simulink model "case6"  (R2024b)
settings: Solver=FixedStepAuto  StartTime=0  StopTime=1  FixedStep=1e-7  RelTol=1e-3
values from neighbouring files (symbols this model uses):
  SG_D_1_D = 0.01056    [IEEE9_case_parameters.m]    (also in case1_parameters.m; case2_parameters.m; case3_parameters.m; case4_parameters.m)
  SG_D_1_EnableSaturation = 0    [IEEE9_case_parameters.m]    (also in case1_parameters.m; case2_parameters.m; case3_parameters.m; case4_parameters.m)
  SG_D_1_f0 = 60    [IEEE9_case_parameters.m]    (also in case1_parameters.m; case2_parameters.m; case3_parameters.m; case4_parameters.m)
  SG_D_1_H = 7.5    [IEEE9_case_parameters.m]    (also in case1_parameters.m; case2_parameters.m; case3_parameters.m; case4_parameters.m)
  SG_D_1_K_A = 20    [IEEE9_case_parameters.m]    (also in case1_parameters.m; case2_parameters.m; case3_parameters.m; case4_parameters.m)
  SG_D_1_K_E = 1.000000e+1    (= 10)    [IEEE9_case_parameters.m]    (also in case1_parameters.m; case2_parameters.m; case3_parameters.m; case4_parameters.m)
  SG_D_1_K_F = 2.363    [IEEE9_case_parameters.m]    (also in case1_parameters.m; case2_parameters.m; case3_parameters.m; case4_parameters.m)
  SG_D_1_K_s = 0.5    [IEEE9_case_parameters.m]    (also in case1_parameters.m = 5; case2_parameters.m = 5; case3_parameters.m = 5; case4_parameters.m = 5)
  SG_D_1_R_a = 0.001088    [IEEE9_case_parameters.m]    (also in case1_parameters.m; case2_parameters.m; case3_parameters.m; case4_parameters.m)
  SG_D_1_S_A = 1    [IEEE9_case_parameters.m]    (also in case1_parameters.m; case2_parameters.m; case3_parameters.m; case4_parameters.m)
  SG_D_1_S_B = 0.103    [IEEE9_case_parameters.m]    (also in case1_parameters.m; case2_parameters.m; case3_parameters.m; case4_parameters.m)
  SG_D_1_S_N = 10.659857    [IEEE9_case_parameters.m]    (also in case1_parameters.m; case2_parameters.m; case3_parameters.m; case4_parameters.m)
  SG_D_1_SpeedPara = 200    [IEEE9_case_parameters.m]    (also in case1_parameters.m; case2_parameters.m; case3_parameters.m; case4_parameters.m)
  SG_D_1_T_0 = 0.720173    [IEEE9_case_parameters.m]    (also in case1_parameters.m = 0.755522; case2_parameters.m = 0.808931; case3_parameters.m = 0.869402; case4_parameters.m = 0.729316)
  SG_D_1_T_1 = 0.3    [IEEE9_case_parameters.m]    (also in case1_parameters.m; case2_parameters.m; case3_parameters.m; case4_parameters.m)
  SG_D_1_T_2 = 0.05    [IEEE9_case_parameters.m]    (also in case1_parameters.m; case2_parameters.m; case3_parameters.m; case4_parameters.m)
  SG_D_1_T_3 = 0.02    [IEEE9_case_parameters.m]    (also in case1_parameters.m; case2_parameters.m; case3_parameters.m; case4_parameters.m)
  SG_D_1_T_4 = 0.005    [IEEE9_case_parameters.m]    (also in case1_parameters.m; case2_parameters.m; case3_parameters.m; case4_parameters.m)
  SG_D_1_T_A = 0.02    [IEEE9_case_parameters.m]    (also in case1_parameters.m; case2_parameters.m; case3_parameters.m; case4_parameters.m)
  SG_D_1_T_dd = 8.000000e+0    (= 8)    [IEEE9_case_parameters.m]    (also in case1_parameters.m; case2_parameters.m; case3_parameters.m; case4_parameters.m)
  SG_D_1_T_ddd = 0.04    [IEEE9_case_parameters.m]    (also in case1_parameters.m; case2_parameters.m; case3_parameters.m; case4_parameters.m)
  SG_D_1_T_E = 0.314    [IEEE9_case_parameters.m]    (also in case1_parameters.m; case2_parameters.m; case3_parameters.m; case4_parameters.m)
  SG_D_1_T_F = 0.35    [IEEE9_case_parameters.m]    (also in case1_parameters.m; case2_parameters.m; case3_parameters.m; case4_parameters.m)
  SG_D_1_T_qd = 0.8    [IEEE9_case_parameters.m]    (also in case1_parameters.m; case2_parameters.m; case3_parameters.m; case4_parameters.m)
  SG_D_1_T_qdd = 0.02    [IEEE9_case_parameters.m]    (also in case1_parameters.m; case2_parameters.m; case3_parameters.m; case4_parameters.m)
  SG_D_1_T_speed = 0.1    [IEEE9_case_parameters.m]    (also in case1_parameters.m = 200; case2_parameters.m = 200; case3_parameters.m = 200; case4_parameters.m = 200)
  SG_D_1_T_w = 0.5    [IEEE9_case_parameters.m]    (also in case1_parameters.m; case2_parameters.m; case3_parameters.m; case4_parameters.m)
  SG_D_1_V_ref = 1.990276    [IEEE9_case_parameters.m]    (also in case1_parameters.m = 2.042296; case2_parameters.m = 2.051388; case3_parameters.m = 2.089584; case4_parameters.m = 2.01845)
  SG_D_1_w_ref = 376.991118    [IEEE9_case_parameters.m]    (also in case1_parameters.m; case2_parameters.m; case3_parameters.m; case4_parameters.m)
  SG_D_1_wb = 6.000000e+1    (= 60)    [IEEE9_case_parameters.m]    (also in case1_parameters.m; case2_parameters.m; case3_parameters.m; case4_parameters.m)
  SG_D_1_x_d = 1.9    [IEEE9_case_parameters.m]    (also in case1_parameters.m; case2_parameters.m; case3_parameters.m; case4_parameters.m)
  SG_D_1_x_dd = 0.302    [IEEE9_case_parameters.m]    (also in case1_parameters.m; case2_parameters.m; case3_parameters.m; case4_parameters.m)
  SG_D_1_x_ddd = 0.204    [IEEE9_case_parameters.m]    (also in case1_parameters.m; case2_parameters.m; case3_parameters.m; case4_parameters.m)
  SG_D_1_x_l = 0.05    [IEEE9_case_parameters.m]    (also in case1_parameters.m; case2_parameters.m; case3_parameters.m; case4_parameters.m)
  SG_D_1_x_q = 1.3    [IEEE9_case_parameters.m]    (also in case1_parameters.m; case2_parameters.m; case3_parameters.m; case4_parameters.m)
  SG_D_1_x_qd = 0.5    [IEEE9_case_parameters.m]    (also in case1_parameters.m; case2_parameters.m; case3_parameters.m; case4_parameters.m)
  SG_D_1_x_qdd = 0.3    [IEEE9_case_parameters.m]    (also in case1_parameters.m; case2_parameters.m; case3_parameters.m; case4_parameters.m)
  SG_D_2_D = 0.02    [IEEE9_case_parameters.m]    (also in case1_parameters.m; case2_parameters.m; case3_parameters.m; case4_parameters.m)
  SG_D_2_EnableSaturation = 0    [IEEE9_case_parameters.m]    (also in case1_parameters.m; case2_parameters.m; case3_parameters.m; case4_parameters.m)
  SG_D_2_f0 = 60    [IEEE9_case_parameters.m]    (also in case1_parameters.m; case2_parameters.m; case3_parameters.m; case4_parameters.m)
  SG_D_2_H = 8.000000e+0    (= 8)    [IEEE9_case_parameters.m]    (also in case1_parameters.m; case2_parameters.m; case3_parameters.m; case4_parameters.m)
  SG_D_2_K_A = 20    [IEEE9_case_parameters.m]    (also in case1_parameters.m; case2_parameters.m; case3_parameters.m; case4_parameters.m)
  SG_D_2_K_E = 1.000000e+1    (= 10)    [IEEE9_case_parameters.m]    (also in case1_parameters.m; case2_parameters.m; case3_parameters.m; case4_parameters.m)
  SG_D_2_K_F = 2.363    [IEEE9_case_parameters.m]    (also in case1_parameters.m; case2_parameters.m; case3_parameters.m; case4_parameters.m)
  SG_D_2_K_s = 0.5    [IEEE9_case_parameters.m]    (also in case1_parameters.m = 4; case2_parameters.m = 4; case3_parameters.m = 4; case4_parameters.m = 4)
  SG_D_2_R_a = 0.001088    [IEEE9_case_parameters.m]    (also in case1_parameters.m; case2_parameters.m; case3_parameters.m; case4_parameters.m)
  SG_D_2_S_A = 1    [IEEE9_case_parameters.m]    (also in case1_parameters.m; case2_parameters.m; case3_parameters.m; case4_parameters.m)
  SG_D_2_S_B = 0.103    [IEEE9_case_parameters.m]    (also in case1_parameters.m; case2_parameters.m; case3_parameters.m; case4_parameters.m)
  SG_D_2_S_N = 10.659857    [IEEE9_case_parameters.m]    (also in case1_parameters.m; case2_parameters.m; case3_parameters.m; case4_parameters.m)
  SG_D_2_SpeedPara = 200    [IEEE9_case_parameters.m]    (also in case1_parameters.m; case2_parameters.m; case3_parameters.m; case4_parameters.m)
  SG_D_2_T_0 = 1.632913    [IEEE9_case_parameters.m]    (also in case1_parameters.m = 1.632925; case2_parameters.m = 1.632915; case3_parameters.m = 1.632914; case4_parameters.m = 1.632927)
  SG_D_2_T_1 = 0.2    [IEEE9_case_parameters.m]    (also in case1_parameters.m; case2_parameters.m; case3_parameters.m; case4_parameters.m)
  SG_D_2_T_2 = 0.05    [IEEE9_case_parameters.m]    (also in case1_parameters.m; case2_parameters.m; case3_parameters.m; case4_parameters.m)
  SG_D_2_T_3 = 0.02    [IEEE9_case_parameters.m]    (also in case1_parameters.m; case2_parameters.m; case3_parameters.m; case4_parameters.m)
  SG_D_2_T_4 = 0.005    [IEEE9_case_parameters.m]    (also in case1_parameters.m; case2_parameters.m; case3_parameters.m; case4_parameters.m)
  SG_D_2_T_A = 0.02    [IEEE9_case_parameters.m]    (also in case1_parameters.m; case2_parameters.m; case3_parameters.m; case4_parameters.m)
  SG_D_2_T_dd = 7.9    [IEEE9_case_parameters.m]    (also in case1_parameters.m; case2_parameters.m; case3_parameters.m; case4_parameters.m)
  SG_D_2_T_ddd = 0.04    [IEEE9_case_parameters.m]    (also in case1_parameters.m; case2_parameters.m; case3_parameters.m; case4_parameters.m)
  SG_D_2_T_E = 0.314    [IEEE9_case_parameters.m]    (also in case1_parameters.m; case2_parameters.m; case3_parameters.m; case4_parameters.m)
  SG_D_2_T_F = 0.35    [IEEE9_case_parameters.m]    (also in case1_parameters.m; case2_parameters.m; case3_parameters.m; case4_parameters.m)
  SG_D_2_T_qd = 0.8    [IEEE9_case_parameters.m]    (also in case1_parameters.m; case2_parameters.m; case3_parameters.m; case4_parameters.m)
  SG_D_2_T_qdd = 0.015    [IEEE9_case_parameters.m]    (also in case1_parameters.m; case2_parameters.m; case3_parameters.m; case4_parameters.m)
  SG_D_2_T_speed = 0.1    [IEEE9_case_parameters.m]    (also in case1_parameters.m = 150; case2_parameters.m = 150; case3_parameters.m = 150; case4_parameters.m = 150)
  SG_D_2_T_w = 0.35    [IEEE9_case_parameters.m]    (also in case1_parameters.m; case2_parameters.m; case3_parameters.m; case4_parameters.m)
  SG_D_2_V_ref = 2.58547    [IEEE9_case_parameters.m]    (also in case1_parameters.m = 2.597896; case2_parameters.m = 2.587136; case3_parameters.m = 2.586042; case4_parameters.m = 2.599679)
  SG_D_2_w_ref = 376.991118    [IEEE9_case_parameters.m]    (also in case1_parameters.m; case2_parameters.m; case3_parameters.m; case4_parameters.m)
  SG_D_2_wb = 6.000000e+1    (= 60)    [IEEE9_case_parameters.m]    (also in case1_parameters.m; case2_parameters.m; case3_parameters.m; case4_parameters.m)
  SG_D_2_x_d = 1.8    [IEEE9_case_parameters.m]    (also in case1_parameters.m; case2_parameters.m; case3_parameters.m; case4_parameters.m)
  SG_D_2_x_dd = 0.302    [IEEE9_case_parameters.m]    (also in case1_parameters.m; case2_parameters.m; case3_parameters.m; case4_parameters.m)
  SG_D_2_x_ddd = 0.204    [IEEE9_case_parameters.m]    (also in case1_parameters.m; case2_parameters.m; case3_parameters.m; case4_parameters.m)
  SG_D_2_x_l = 0.05    [IEEE9_case_parameters.m]    (also in case1_parameters.m; case2_parameters.m; case3_parameters.m; case4_parameters.m)
  SG_D_2_x_q = 1.25    [IEEE9_case_parameters.m]    (also in case1_parameters.m; case2_parameters.m; case3_parameters.m; case4_parameters.m)
  SG_D_2_x_qd = 0.5    [IEEE9_case_parameters.m]    (also in case1_parameters.m; case2_parameters.m; case3_parameters.m; case4_parameters.m)
  SG_D_2_x_qdd = 0.3    [IEEE9_case_parameters.m]    (also in case1_parameters.m; case2_parameters.m; case3_parameters.m; case4_parameters.m)
  SG_D_3_D = 0.02    [IEEE9_case_parameters.m]    (also in case1_parameters.m; case2_parameters.m; case3_parameters.m; case4_parameters.m)
  SG_D_3_EnableSaturation = 0    [IEEE9_case_parameters.m]    (also in case1_parameters.m; case2_parameters.m; case3_parameters.m; case4_parameters.m)
  SG_D_3_f0 = 60    [IEEE9_case_parameters.m]    (also in case1_parameters.m; case2_parameters.m; case3_parameters.m; case4_parameters.m)
  SG_D_3_H = 7.7    [IEEE9_case_parameters.m]    (also in case1_parameters.m; case2_parameters.m; case3_parameters.m; case4_parameters.m)
  SG_D_3_K_A = 20    [IEEE9_case_parameters.m]    (also in case1_parameters.m; case2_parameters.m; case3_parameters.m; case4_parameters.m)
  SG_D_3_K_E = 1.000000e+1    (= 10)    [IEEE9_case_parameters.m]    (also in case1_parameters.m; case2_parameters.m; case3_parameters.m; case4_parameters.m)
  SG_D_3_K_F = 2.363    [IEEE9_case_parameters.m]    (also in case1_parameters.m; case2_parameters.m; case3_parameters.m; case4_parameters.m)
  SG_D_3_K_s = 0.2    [IEEE9_case_parameters.m]    (also in case1_parameters.m = 2; case2_parameters.m = 2; case3_parameters.m = 2; case4_parameters.m = 2)
  SG_D_3_R_a = 0.001088    [IEEE9_case_parameters.m]    (also in case1_parameters.m; case2_parameters.m; case3_parameters.m; case4_parameters.m)
  SG_D_3_S_A = 1    [IEEE9_case_parameters.m]    (also in case1_parameters.m; case2_parameters.m; case3_parameters.m; case4_parameters.m)
  SG_D_3_S_B = 0.103    [IEEE9_case_parameters.m]    (also in case1_parameters.m; case2_parameters.m; case3_parameters.m; case4_parameters.m)
  SG_D_3_S_N = 10.659857    [IEEE9_case_parameters.m]    (also in case1_parameters.m; case2_parameters.m; case3_parameters.m; case4_parameters.m)
  SG_D_3_SpeedPara = 200    [IEEE9_case_parameters.m]    (also in case1_parameters.m; case2_parameters.m; case3_parameters.m; case4_parameters.m)
  SG_D_3_T_0 = 0.850788    [IEEE9_case_parameters.m]    (also in case1_parameters.m = 0.850786; case2_parameters.m = 0.850787; case3_parameters.m; case4_parameters.m = 0.850786)
  SG_D_3_T_1 = 0.2    [IEEE9_case_parameters.m]    (also in case1_parameters.m; case2_parameters.m; case3_parameters.m; case4_parameters.m)
  SG_D_3_T_2 = 0.05    [IEEE9_case_parameters.m]    (also in case1_parameters.m; case2_parameters.m; case3_parameters.m; case4_parameters.m)
  SG_D_3_T_3 = 0.02    [IEEE9_case_parameters.m]    (also in case1_parameters.m; case2_parameters.m; case3_parameters.m; case4_parameters.m)
  SG_D_3_T_4 = 0.005    [IEEE9_case_parameters.m]    (also in case1_parameters.m; case2_parameters.m; case3_parameters.m; case4_parameters.m)
  SG_D_3_T_A = 0.02    [IEEE9_case_parameters.m]    (also in case1_parameters.m; case2_parameters.m; case3_parameters.m; case4_parameters.m)
  SG_D_3_T_dd = 8.1    [IEEE9_case_parameters.m]    (also in case1_parameters.m; case2_parameters.m; case3_parameters.m; case4_parameters.m)
  SG_D_3_T_ddd = 0.04    [IEEE9_case_parameters.m]    (also in case1_parameters.m; case2_parameters.m; case3_parameters.m; case4_parameters.m)
  SG_D_3_T_E = 0.314    [IEEE9_case_parameters.m]    (also in case1_parameters.m; case2_parameters.m; case3_parameters.m; case4_parameters.m)
  SG_D_3_T_F = 0.35    [IEEE9_case_parameters.m]    (also in case1_parameters.m; case2_parameters.m; case3_parameters.m; case4_parameters.m)
  SG_D_3_T_qd = 0.8    [IEEE9_case_parameters.m]    (also in case1_parameters.m; case2_parameters.m; case3_parameters.m; case4_parameters.m)
  SG_D_3_T_qdd = 0.015    [IEEE9_case_parameters.m]    (also in case1_parameters.m; case2_parameters.m; case3_parameters.m; case4_parameters.m)
  SG_D_3_T_speed = 0.1    [IEEE9_case_parameters.m]    (also in case1_parameters.m = 180; case2_parameters.m = 180; case3_parameters.m = 180; case4_parameters.m = 180)
  SG_D_3_T_w = 0.4    [IEEE9_case_parameters.m]    (also in case1_parameters.m; case2_parameters.m; case3_parameters.m; case4_parameters.m)
  SG_D_3_V_ref = 1.892727    [IEEE9_case_parameters.m]    (also in case1_parameters.m = 1.906439; case2_parameters.m = 1.895535; case3_parameters.m = 1.892105; case4_parameters.m = 1.906598)
  SG_D_3_w_ref = 376.991118    [IEEE9_case_parameters.m]    (also in case1_parameters.m; case2_parameters.m; case3_parameters.m; case4_parameters.m)
  SG_D_3_wb = 6.000000e+1    (= 60)    [IEEE9_case_parameters.m]    (also in case1_parameters.m; case2_parameters.m; case3_parameters.m; case4_parameters.m)
  SG_D_3_x_d = 1.85    [IEEE9_case_parameters.m]    (also in case1_parameters.m; case2_parameters.m; case3_parameters.m; case4_parameters.m)
  SG_D_3_x_dd = 0.302    [IEEE9_case_parameters.m]    (also in case1_parameters.m; case2_parameters.m; case3_parameters.m; case4_parameters.m)
  SG_D_3_x_ddd = 0.204    [IEEE9_case_parameters.m]    (also in case1_parameters.m; case2_parameters.m; case3_parameters.m; case4_parameters.m)
  SG_D_3_x_l = 0.05    [IEEE9_case_parameters.m]    (also in case1_parameters.m; case2_parameters.m; case3_parameters.m; case4_parameters.m)
  SG_D_3_x_q = 1.2    [IEEE9_case_parameters.m]    (also in case1_parameters.m; case2_parameters.m; case3_parameters.m; case4_parameters.m)
  SG_D_3_x_qd = 0.5    [IEEE9_case_parameters.m]    (also in case1_parameters.m; case2_parameters.m; case3_parameters.m; case4_parameters.m)
  SG_D_3_x_qdd = 0.3    [IEEE9_case_parameters.m]    (also in case1_parameters.m; case2_parameters.m; case3_parameters.m; case4_parameters.m)
(part 4 of 12)

== system case6/AC_1/d_vq_bus_7_block ==
  note: d_vq_bus_7 in case6
      | $2106.09563369148\,\mathrm{iq}_{\mathrm{bus},7}-376.991118430775\,\mathrm{vd}_{\mathrm{bus},7}$
      | Automatically generated on 2025-10-31 19:20:33 .
  Alge_iq_bus_7_2005b : Inport
  State_vd_bus_7_eb09d : Inport  Port=2
  Constant_2106.09563369148_078d3 : Constant  Value=2106.09563369148
  Constant_376.991118430775_d6c8b : Constant  Value=376.991118430775
  Product_5f1c9 : Product
  Product_e99b3 : Product
  Subtract_9b446 : Sum  Inputs=+-
  Blockout_d_vq_bus_7_5af5d : Outport
  wires:
  Constant_2106.09563369148_078d3/1 -> Product_e99b3/1
  Product_5f1c9/1 -> Subtract_9b446/2
  Alge_iq_bus_7_2005b/1 -> Product_e99b3/2
  Constant_376.991118430775_d6c8b/1 -> Product_5f1c9/1
  Subtract_9b446/1 -> Blockout_d_vq_bus_7_5af5d/1
  State_vd_bus_7_eb09d/1 -> Product_5f1c9/2
  Product_e99b3/1 -> Subtract_9b446/1

== system case6/AC_1/d_vq_bus_8_block ==
  note: d_vq_bus_8 in case6
      | $1657.10381727813\,\mathrm{iq}_{\mathrm{bus},8}-376.991118430775\,\mathrm{vd}_{\mathrm{bus},8}$
      | Automatically generated on 2025-10-31 19:20:35 .
  Alge_iq_bus_8_f5035 : Inport
  State_vd_bus_8_bd411 : Inport  Port=2
  Constant_1657.10381727813_ce04b : Constant  Value=1657.10381727813
  Constant_376.991118430775_359d2 : Constant  Value=376.991118430775
  Product_21817 : Product
  Product_6201e : Product
  Subtract_2f806 : Sum  Inputs=+-
  Blockout_d_vq_bus_8_43ab1 : Outport
  wires:
  Constant_1657.10381727813_ce04b/1 -> Product_6201e/1
  Constant_376.991118430775_359d2/1 -> Product_21817/1
  Alge_iq_bus_8_f5035/1 -> Product_6201e/2
  State_vd_bus_8_bd411/1 -> Product_21817/2
  Product_6201e/1 -> Subtract_2f806/1
  Product_21817/1 -> Subtract_2f806/2
  Subtract_2f806/1 -> Blockout_d_vq_bus_8_43ab1/1

== system case6/AC_1/d_vq_bus_9_block ==
  note: d_vq_bus_9 in case6
      | $1564.27849971276\,\mathrm{iq}_{\mathrm{bus},9}-376.991118430775\,\mathrm{vd}_{\mathrm{bus},9}$
      | Automatically generated on 2025-10-31 19:20:37 .
  Alge_iq_bus_9_635a6 : Inport
  State_vd_bus_9_01655 : Inport  Port=2
  Constant_1564.27849971276_91bb5 : Constant  Value=1564.27849971276
  Constant_376.991118430775_72151 : Constant  Value=376.991118430775
  Product_87976 : Product
  Product_b87c1 : Product
  Subtract_a505a : Sum  Inputs=+-
  Blockout_d_vq_bus_9_b4666 : Outport
  wires:
  Constant_1564.27849971276_91bb5/1 -> Product_87976/1
  Constant_376.991118430775_72151/1 -> Product_b87c1/1
  Alge_iq_bus_9_635a6/1 -> Product_87976/2
  State_vd_bus_9_01655/1 -> Product_b87c1/2
  Product_87976/1 -> Subtract_a505a/1
  Product_b87c1/1 -> Subtract_a505a/2
  Subtract_a505a/1 -> Blockout_d_vq_bus_9_b4666/1

== system case6/AC_1/id_bus_1_block ==
  note: id_bus_1 in case6
      | $\mathrm{id}_{\mathrm{SG},D,1}-\mathrm{id}_{\mathrm{line},1,4}$
      | Automatically generated on 2025-10-31 19:21:17 .
  Input_id_SG_D_1_1909b : Inport
  State_id_line_1_4_cba7d : Inport  Port=2
  Subtract_f9eb5 : Sum  Inputs=+-
  Blockout_id_bus_1_b268c : Outport
  wires:
  Input_id_SG_D_1_1909b/1 -> Subtract_f9eb5/1
  State_id_line_1_4_cba7d/1 -> Subtract_f9eb5/2
  Subtract_f9eb5/1 -> Blockout_id_bus_1_b268c/1

== system case6/AC_1/id_bus_2_block ==
  note: id_bus_2 in case6
      | $\mathrm{id}_{\mathrm{SG},D,2}+\mathrm{id}_{\mathrm{line},8,2}$
      | Automatically generated on 2025-10-31 19:21:20 .
  Input_id_SG_D_2_3ebd4 : Inport
  State_id_line_8_2_f66c5 : Inport  Port=2
  Add_0372f : Sum
  Blockout_id_bus_2_4fb07 : Outport
  wires:
  Input_id_SG_D_2_3ebd4/1 -> Add_0372f/1
  State_id_line_8_2_f66c5/1 -> Add_0372f/2
  Add_0372f/1 -> Blockout_id_bus_2_4fb07/1

== system case6/AC_1/id_bus_3_block ==
  note: id_bus_3 in case6
      | $\mathrm{id}_{\mathrm{SG},D,3}-\mathrm{id}_{\mathrm{line},3,6}$
      | Automatically generated on 2025-10-31 19:21:22 .
  Input_id_SG_D_3_f42f9 : Inport
  State_id_line_3_6_8a779 : Inport  Port=2
  Subtract_84151 : Sum  Inputs=+-
  Blockout_id_bus_3_89124 : Outport
  wires:
  Input_id_SG_D_3_f42f9/1 -> Subtract_84151/1
  State_id_line_3_6_8a779/1 -> Subtract_84151/2
  Subtract_84151/1 -> Blockout_id_bus_3_89124/1

== system case6/AC_1/id_bus_4_block ==
  note: id_bus_4 in case6
      | $\mathrm{id}_{\mathrm{line},1,4}-\mathrm{id}_{\mathrm{line},4,5}+\mathrm{id}_{\mathrm{line},9,4}$
      | Automatically generated on 2025-10-31 19:21:24 .
  State_id_line_1_4_a2627 : Inport
  State_id_line_4_5_a6682 : Inport  Port=2
  State_id_line_9_4_09bfd : Inport  Port=3
  Add_27027 : Sum
  Subtract_43973 : Sum  Inputs=+-
  Blockout_id_bus_4_ca704 : Outport
  wires:
  State_id_line_9_4_09bfd/1 -> Add_27027/2
  State_id_line_1_4_a2627/1 -> Subtract_43973/1
  State_id_line_4_5_a6682/1 -> Subtract_43973/2
  Subtract_43973/1 -> Add_27027/1
  Add_27027/1 -> Blockout_id_bus_4_ca704/1

== system case6/AC_1/id_bus_5_block ==
  note: id_bus_5 in case6
      | $\mathrm{id}_{\mathrm{line},4,5}-\mathrm{id}_{\mathrm{load},5}-\mathrm{id}_{\mathrm{line},5,6}$
      | Automatically generated on 2025-10-31 19:21:26 .
  State_id_load_5_e4a9a : Inport
  State_id_line_4_5_d68f5 : Inport  Port=2
  State_id_line_5_6_d8d07 : Inport  Port=3
  Add_41afa : Sum
  Constant_-1_afe1f : Constant  Value=-1
  Product_c93ba : Product
  Subtract_799f6 : Sum  Inputs=+-
  Blockout_id_bus_5_39616 : Outport
  wires:
  Subtract_799f6/1 -> Blockout_id_bus_5_39616/1
  State_id_line_4_5_d68f5/1 -> Add_41afa/2
  Constant_-1_afe1f/1 -> Product_c93ba/1
  Add_41afa/1 -> Subtract_799f6/1
  State_id_load_5_e4a9a/1 -> Product_c93ba/2
  Product_c93ba/1 -> Add_41afa/1
  State_id_line_5_6_d8d07/1 -> Subtract_799f6/2

== system case6/AC_1/id_bus_6_block ==
  note: id_bus_6 in case6
      | $\mathrm{id}_{\mathrm{line},3,6}+\mathrm{id}_{\mathrm{line},5,6}-\mathrm{id}_{\mathrm{line},6,7}$
      | Automatically generated on 2025-10-31 19:21:28 .
  State_id_line_3_6_9e91b : Inport
  State_id_line_5_6_fe13e : Inport  Port=2
  State_id_line_6_7_6b30b : Inport  Port=3
  Add_465c7 : Sum
  Subtract_d54d8 : Sum  Inputs=+-
  Blockout_id_bus_6_f0019 : Outport
  wires:
  State_id_line_6_7_6b30b/1 -> Subtract_d54d8/2
  State_id_line_3_6_9e91b/1 -> Add_465c7/1
  State_id_line_5_6_fe13e/1 -> Add_465c7/2
  Add_465c7/1 -> Subtract_d54d8/1
  Subtract_d54d8/1 -> Blockout_id_bus_6_f0019/1

== system case6/AC_1/id_bus_7_block ==
  note: id_bus_7 in case6
      | $\mathrm{id}_{\mathrm{line},6,7}-\mathrm{id}_{\mathrm{load},7}-\mathrm{id}_{\mathrm{line},7,8}$
      | Automatically generated on 2025-10-31 19:21:30 .
  State_id_load_7_33856 : Inport
  State_id_line_6_7_91e84 : Inport  Port=2
  State_id_line_7_8_65e8d : Inport  Port=3
  Add_e3068 : Sum
  Constant_-1_4fccf : Constant  Value=-1
  Product_24095 : Product
  Subtract_30b93 : Sum  Inputs=+-
  Blockout_id_bus_7_0b458 : Outport
  wires:
  Subtract_30b93/1 -> Blockout_id_bus_7_0b458/1
  State_id_line_6_7_91e84/1 -> Add_e3068/2
  Constant_-1_4fccf/1 -> Product_24095/1
  Add_e3068/1 -> Subtract_30b93/1
  State_id_load_7_33856/1 -> Product_24095/2
  Product_24095/1 -> Add_e3068/1
  State_id_line_7_8_65e8d/1 -> Subtract_30b93/2

== system case6/AC_1/id_bus_8_block ==
  note: id_bus_8 in case6
      | $\mathrm{id}_{\mathrm{line},7,8}-\mathrm{id}_{\mathrm{line},8,2}-\mathrm{id}_{\mathrm{line},8,9}$
      | Automatically generated on 2025-10-31 19:21:32 .
  State_id_line_7_8_6dd2f : Inport
  State_id_line_8_2_e60f9 : Inport  Port=2
  State_id_line_8_9_45767 : Inport  Port=3
  Subtract_13a15 : Sum  Inputs=+-
  Subtract_15c8a : Sum  Inputs=+-
  Blockout_id_bus_8_eda9d : Outport
  wires:
  State_id_line_8_9_45767/1 -> Subtract_15c8a/2
  State_id_line_7_8_6dd2f/1 -> Subtract_13a15/1
  State_id_line_8_2_e60f9/1 -> Subtract_13a15/2
  Subtract_13a15/1 -> Subtract_15c8a/1
  Subtract_15c8a/1 -> Blockout_id_bus_8_eda9d/1

== system case6/AC_1/id_bus_9_block ==
  note: id_bus_9 in case6
      | $\mathrm{id}_{\mathrm{line},8,9}-\mathrm{id}_{\mathrm{load},9}-\mathrm{id}_{\mathrm{line},9,4}$
      | Automatically generated on 2025-10-31 19:21:34 .
  State_id_load_9_96b66 : Inport
  State_id_line_8_9_df04e : Inport  Port=2
  State_id_line_9_4_02d88 : Inport  Port=3
  Add_5ffc7 : Sum
  Constant_-1_72ba1 : Constant  Value=-1
  Product_2e360 : Product
  Subtract_3b0e8 : Sum  Inputs=+-
  Blockout_id_bus_9_51cea : Outport
  wires:
  Subtract_3b0e8/1 -> Blockout_id_bus_9_51cea/1
  State_id_line_8_9_df04e/1 -> Add_5ffc7/2
  Constant_-1_72ba1/1 -> Product_2e360/1
  Add_5ffc7/1 -> Subtract_3b0e8/1
  State_id_load_9_96b66/1 -> Product_2e360/2
  Product_2e360/1 -> Add_5ffc7/1
  State_id_line_9_4_02d88/1 -> Subtract_3b0e8/2

== system case6/AC_1/iq_bus_1_block ==
  note: iq_bus_1 in case6
      | $\mathrm{iq}_{\mathrm{SG},D,1}-\mathrm{iq}_{\mathrm{line},1,4}$
      | Automatically generated on 2025-10-31 19:21:17 .
  Input_iq_SG_D_1_c869a : Inport
  State_iq_line_1_4_4f8d0 : Inport  Port=2
  Subtract_68c00 : Sum  Inputs=+-
  Blockout_iq_bus_1_c5112 : Outport
  wires:
  Input_iq_SG_D_1_c869a/1 -> Subtract_68c00/1
  State_iq_line_1_4_4f8d0/1 -> Subtract_68c00/2
  Subtract_68c00/1 -> Blockout_iq_bus_1_c5112/1

== system case6/AC_1/iq_bus_2_block ==
  note: iq_bus_2 in case6
      | $\mathrm{iq}_{\mathrm{SG},D,2}+\mathrm{iq}_{\mathrm{line},8,2}$
      | Automatically generated on 2025-10-31 19:21:20 .
  Input_iq_SG_D_2_471fc : Inport
  State_iq_line_8_2_e8e09 : Inport  Port=2
  Add_4be8f : Sum
  Blockout_iq_bus_2_f1d15 : Outport
  wires:
  Input_iq_SG_D_2_471fc/1 -> Add_4be8f/1
  State_iq_line_8_2_e8e09/1 -> Add_4be8f/2
  Add_4be8f/1 -> Blockout_iq_bus_2_f1d15/1

== system case6/AC_1/iq_bus_3_block ==
  note: iq_bus_3 in case6
      | $\mathrm{iq}_{\mathrm{SG},D,3}-\mathrm{iq}_{\mathrm{line},3,6}$
      | Automatically generated on 2025-10-31 19:21:23 .
  Input_iq_SG_D_3_c9bea : Inport
  State_iq_line_3_6_b8aac : Inport  Port=2
  Subtract_5d684 : Sum  Inputs=+-
  Blockout_iq_bus_3_54a2d : Outport
  wires:
  Input_iq_SG_D_3_c9bea/1 -> Subtract_5d684/1
  State_iq_line_3_6_b8aac/1 -> Subtract_5d684/2
  Subtract_5d684/1 -> Blockout_iq_bus_3_54a2d/1

== system case6/AC_1/iq_bus_4_block ==
  note: iq_bus_4 in case6
      | $\mathrm{iq}_{\mathrm{line},1,4}-\mathrm{iq}_{\mathrm{line},4,5}+\mathrm{iq}_{\mathrm{line},9,4}$
      | Automatically generated on 2025-10-31 19:21:25 .
  State_iq_line_1_4_0b9d2 : Inport
  State_iq_line_4_5_235e1 : Inport  Port=2
  State_iq_line_9_4_e6964 : Inport  Port=3
  Add_0496e : Sum
  Subtract_90f4d : Sum  Inputs=+-
  Blockout_iq_bus_4_aea66 : Outport
  wires:
  State_iq_line_1_4_0b9d2/1 -> Subtract_90f4d/1
  State_iq_line_4_5_235e1/1 -> Subtract_90f4d/2
  Subtract_90f4d/1 -> Add_0496e/1
  State_iq_line_9_4_e6964/1 -> Add_0496e/2
  Add_0496e/1 -> Blockout_iq_bus_4_aea66/1

== system case6/AC_1/iq_bus_5_block ==
  note: iq_bus_5 in case6
      | $\mathrm{iq}_{\mathrm{line},4,5}-\mathrm{iq}_{\mathrm{load},5}-\mathrm{iq}_{\mathrm{line},5,6}$
      | Automatically generated on 2025-10-31 19:21:27 .
  State_iq_load_5_a48ab : Inport
  State_iq_line_4_5_75c3a : Inport  Port=2
  State_iq_line_5_6_da04c : Inport  Port=3
  Add_85a21 : Sum
  Constant_-1_4a4e3 : Constant  Value=-1
  Product_911f1 : Product
  Subtract_66ccf : Sum  Inputs=+-
  Blockout_iq_bus_5_b826b : Outport
  wires:
  Subtract_66ccf/1 -> Blockout_iq_bus_5_b826b/1
  State_iq_line_4_5_75c3a/1 -> Add_85a21/2
  Constant_-1_4a4e3/1 -> Product_911f1/1
  State_iq_load_5_a48ab/1 -> Product_911f1/2
  Product_911f1/1 -> Add_85a21/1
  Add_85a21/1 -> Subtract_66ccf/1
  State_iq_line_5_6_da04c/1 -> Subtract_66ccf/2

== system case6/AC_1/iq_bus_6_block ==
  note: iq_bus_6 in case6
      | $\mathrm{iq}_{\mathrm{line},3,6}+\mathrm{iq}_{\mathrm{line},5,6}-\mathrm{iq}_{\mathrm{line},6,7}$
      | Automatically generated on 2025-10-31 19:21:29 .
  State_iq_line_3_6_6c42b : Inport
  State_iq_line_5_6_a2426 : Inport  Port=2
  State_iq_line_6_7_fbd66 : Inport  Port=3
  Add_1fb5d : Sum
  Subtract_c939b : Sum  Inputs=+-
  Blockout_iq_bus_6_6aaed : Outport
  wires:
  State_iq_line_3_6_6c42b/1 -> Add_1fb5d/1
  State_iq_line_5_6_a2426/1 -> Add_1fb5d/2
  Add_1fb5d/1 -> Subtract_c939b/1
  State_iq_line_6_7_fbd66/1 -> Subtract_c939b/2
  Subtract_c939b/1 -> Blockout_iq_bus_6_6aaed/1

== system case6/AC_1/iq_bus_7_block ==
  note: iq_bus_7 in case6
      | $\mathrm{iq}_{\mathrm{line},6,7}-\mathrm{iq}_{\mathrm{load},7}-\mathrm{iq}_{\mathrm{line},7,8}$
      | Automatically generated on 2025-10-31 19:21:31 .
  State_iq_load_7_fd394 : Inport
  State_iq_line_6_7_889cc : Inport  Port=2
  State_iq_line_7_8_c812c : Inport  Port=3
  Add_7283f : Sum
  Constant_-1_86704 : Constant  Value=-1
  Product_d3b4a : Product
  Subtract_4b14d : Sum  Inputs=+-
  Blockout_iq_bus_7_c0161 : Outport
  wires:
  Subtract_4b14d/1 -> Blockout_iq_bus_7_c0161/1
  State_iq_line_6_7_889cc/1 -> Add_7283f/2
  Constant_-1_86704/1 -> Product_d3b4a/1
  State_iq_load_7_fd394/1 -> Product_d3b4a/2
  Product_d3b4a/1 -> Add_7283f/1
  Add_7283f/1 -> Subtract_4b14d/1
  State_iq_line_7_8_c812c/1 -> Subtract_4b14d/2

== system case6/AC_1/iq_bus_8_block ==
  note: iq_bus_8 in case6
      | $\mathrm{iq}_{\mathrm{line},7,8}-\mathrm{iq}_{\mathrm{line},8,2}-\mathrm{iq}_{\mathrm{line},8,9}$
      | Automatically generated on 2025-10-31 19:21:33 .
  State_iq_line_7_8_13f88 : Inport
  State_iq_line_8_2_2ae52 : Inport  Port=2
  State_iq_line_8_9_0180a : Inport  Port=3
  Subtract_18c1c : Sum  Inputs=+-
  Subtract_7d233 : Sum  Inputs=+-
  Blockout_iq_bus_8_74d80 : Outport
  wires:
  State_iq_line_7_8_13f88/1 -> Subtract_7d233/1
  State_iq_line_8_2_2ae52/1 -> Subtract_7d233/2
  Subtract_7d233/1 -> Subtract_18c1c/1
  State_iq_line_8_9_0180a/1 -> Subtract_18c1c/2
  Subtract_18c1c/1 -> Blockout_iq_bus_8_74d80/1

== system case6/AC_1/iq_bus_9_block ==
  note: iq_bus_9 in case6
      | $\mathrm{iq}_{\mathrm{line},8,9}-\mathrm{iq}_{\mathrm{load},9}-\mathrm{iq}_{\mathrm{line},9,4}$
      | Automatically generated on 2025-10-31 19:21:35 .
  State_iq_load_9_3ff8b : Inport
  State_iq_line_8_9_ad854 : Inport  Port=2
  State_iq_line_9_4_af760 : Inport  Port=3
  Add_59590 : Sum
  Constant_-1_f3d16 : Constant  Value=-1
  Product_6907c : Product
  Subtract_175ce : Sum  Inputs=+-
  Blockout_iq_bus_9_9e11c : Outport
  wires:
  Subtract_175ce/1 -> Blockout_iq_bus_9_9e11c/1
  State_iq_line_8_9_ad854/1 -> Add_59590/2
  Constant_-1_f3d16/1 -> Product_6907c/1
  State_iq_load_9_3ff8b/1 -> Product_6907c/2
  Product_6907c/1 -> Add_59590/1
  Add_59590/1 -> Subtract_175ce/1
  State_iq_line_9_4_af760/1 -> Subtract_175ce/2

== system case6/AC_1/vd_bus_1_out_block ==
  note: vd_bus_1_out in case6
      | $\mathrm{vd}_{\mathrm{bus},1}$
      | Automatically generated on 2025-10-31 19:21:15 .
  State_vd_bus_1_64b20 : Inport
  Blockout_vd_bus_1_out_fd68c : Outport
  wires:
  State_vd_bus_1_64b20/1 -> Blockout_vd_bus_1_out_fd68c/1

== system case6/AC_1/vd_bus_2_out_block ==
  note: vd_bus_2_out in case6
      | $\mathrm{vd}_{\mathrm{bus},2}$
      | Automatically generated on 2025-10-31 19:21:18 .
  State_vd_bus_2_6d8b2 : Inport
  Blockout_vd_bus_2_out_c0c26 : Outport
  wires:
  State_vd_bus_2_6d8b2/1 -> Blockout_vd_bus_2_out_c0c26/1

== system case6/AC_1/vd_bus_3_out_block ==
  note: vd_bus_3_out in case6
      | $\mathrm{vd}_{\mathrm{bus},3}$
      | Automatically generated on 2025-10-31 19:21:21 .
  State_vd_bus_3_58eaf : Inport
  Blockout_vd_bus_3_out_76727 : Outport
  wires:
  State_vd_bus_3_58eaf/1 -> Blockout_vd_bus_3_out_76727/1

== system case6/AC_1/vq_bus_1_out_block ==
  note: vq_bus_1_out in case6
      | $\mathrm{vq}_{\mathrm{bus},1}$
      | Automatically generated on 2025-10-31 19:21:16 .
  State_vq_bus_1_c6ac3 : Inport
  Blockout_vq_bus_1_out_454ab : Outport
  wires:
  State_vq_bus_1_c6ac3/1 -> Blockout_vq_bus_1_out_454ab/1

== system case6/AC_1/vq_bus_2_out_block ==
  note: vq_bus_2_out in case6
      | $\mathrm{vq}_{\mathrm{bus},2}$
      | Automatically generated on 2025-10-31 19:21:19 .
  State_vq_bus_2_90ade : Inport
  Blockout_vq_bus_2_out_9bd8f : Outport
  wires:
  State_vq_bus_2_90ade/1 -> Blockout_vq_bus_2_out_9bd8f/1

== system case6/AC_1/vq_bus_3_out_block ==
  note: vq_bus_3_out in case6
      | $\mathrm{vq}_{\mathrm{bus},3}$
      | Automatically generated on 2025-10-31 19:21:22 .
  State_vq_bus_3_38926 : Inport
  Blockout_vq_bus_3_out_eff6b : Outport
  wires:
  State_vq_bus_3_38926/1 -> Blockout_vq_bus_3_out_eff6b/1

== system case6/SG_D_1/T_e_SG_D_1_block ==
  note: T_e_SG_D_1 in case6
      | $-\frac{\psi _{d,\mathrm{SG},D,1}\,\left(\psi _{q,\mathrm{SG},D,1}+\frac{\psi _{\mathrm{gq},\mathrm{SG},D,1}\,\left(x_{l}-x_{\mathrm{qdd}}\right)}{x_{l}-x_{\mathrm{qd}}}+\frac{\psi _{\mathrm{kq},\mathrm{SG},D,1}\,\left(x_{\mathrm{qd}}-x_{\mathrm{qdd}}\right)}{x_{l}-x_{\mathrm{qd}}}\right)}{x_{\mathrm{qdd}}}-\frac{\psi _{q,\mathrm{SG},D,1}\,\left(\frac{\psi _{\mathrm{1d},\mathrm{SG},D,1}\,\left(x_{\mathrm{dd}}-x_{\mathrm{ddd}}\right)}{x_{\mathrm{dd}}-x_{l}}-\psi _{d,\mathrm{SG},D,1}+\frac{\psi _{\mathrm{fd},\mathrm{SG},D,1}\,\left(x_{\mathrm{ddd}}-x_{l}\right)}{x_{\mathrm{dd}}-x_{l}}\right)}{x_{\mathrm{ddd}}}$
      | Automatically generated on 2025-10-31 19:17:19 .
  State_psi_d_SG_D_1_e2ff8 : Inport
  State_psi_gq_SG_D_1_d9ca3 : Inport  Port=2
  State_psi_kq_SG_D_1_0f8e3 : Inport  Port=3
  State_psi_q_SG_D_1_2f227 : Inport  Port=4
  State_psi_q_SG_D_1_52964 : Inport  Port=5
  State_psi_1d_SG_D_1_f309e : Inport  Port=6
  State_psi_d_SG_D_1_8592d : Inport  Port=7
  State_psi_fd_SG_D_1_d1c10 : Inport  Port=8
  Add_04fe2 : Sum
  Add_41e5d : Sum
  Add_7aebe : Sum
  Add_8b435 : Sum
  Add_b16f4 : Sum
  Add_cd29b : Sum
  Constant_-1_678d3 : Constant  Value=-1
  Constant_-1_b85fd : Constant  Value=-1
  Constant_-1_e4171 : Constant  Value=-1
  Constant_-1_f6887 : Constant  Value=-1
  Constant_-1_fbcda : Constant  Value=-1
  Constant_x_dd_10022 : Constant  Value=x_dd
  Constant_x_dd_31c0f : Constant  Value=x_dd
  Constant_x_dd_bd552 : Constant  Value=x_dd
  Constant_x_ddd_62423 : Constant  Value=x_ddd
  Constant_x_ddd_6a04f : Constant  Value=x_ddd
  Constant_x_ddd_8eddf : Constant  Value=x_ddd
  Constant_x_l_483a0 : Constant  Value=x_l
  Constant_x_l_4baef : Constant  Value=x_l
  Constant_x_l_a8e7e : Constant  Value=x_l
  Constant_x_l_aae67 : Constant  Value=x_l
  Constant_x_l_e8292 : Constant  Value=x_l
  Constant_x_l_fc660 : Constant  Value=x_l
  Constant_x_qd_0e766 : Constant  Value=x_qd
  Constant_x_qd_2b014 : Constant  Value=x_qd
  Constant_x_qd_59921 : Constant  Value=x_qd
  Constant_x_qdd_7b7f5 : Constant  Value=x_qdd
  Constant_x_qdd_a111b : Constant  Value=x_qdd
  Constant_x_qdd_d12bc : Constant  Value=x_qdd
  Divide_2779c : Product  Inputs=*/
  Divide_30c30 : Product  Inputs=*/
  Divide_7cbd0 : Product  Inputs=*/
  Divide_b9c05 : Product  Inputs=*/
  Divide_c5dbb : Product  Inputs=*/
  Divide_f6ea0 : Product  Inputs=*/
  Product_1e13a : Product
  Product_28f44 : Product
  Product_444a5 : Product
  Product_72354 : Product
  Product_90f35 : Product
  Product_9fd1e : Product
  Product_a161f : Product
  Product_aae9b : Product
  Product_b7782 : Product
  Product_c89ea : Product
  Product_f8e2c : Product
  Subtract_16297 : Sum  Inputs=+-
  Subtract_37645 : Sum  Inputs=+-
  Subtract_50a5f : Sum  Inputs=+-
  Subtract_8cdf0 : Sum  Inputs=+-
  Subtract_a62de : Sum  Inputs=+-
  Subtract_c749b : Sum  Inputs=+-
  Subtract_f0ea0 : Sum  Inputs=+-
  Blockout_T_e_SG_D_1_2bf50 : Outport
  wires:
  Product_72354/1 -> Divide_2779c/1
  Product_9fd1e/1 -> Add_8b435/1
  Divide_2779c/1 -> Subtract_c749b/1
  Constant_-1_b85fd/1 -> Product_9fd1e/1
  Constant_x_l_fc660/1 -> Product_9fd1e/2
  Constant_x_qdd_a111b/1 -> Add_8b435/2
  Constant_x_qd_0e766/1 -> Subtract_16297/1
  Constant_-1_e4171/1 -> Product_f8e2c/1
  Constant_x_qdd_7b7f5/1 -> Divide_30c30/2
  Constant_x_qdd_d12bc/1 -> Subtract_16297/2
  State_psi_q_SG_D_1_52964/1 -> Product_1e13a/1
  Constant_x_dd_31c0f/1 -> Subtract_f0ea0/1
  Constant_x_l_483a0/1 -> Product_f8e2c/2
  Subtract_f0ea0/1 -> Product_a161f/2
  Constant_-1_f6887/1 -> Product_28f44/1
  Constant_x_l_e8292/1 -> Product_28f44/2
  Subtract_8cdf0/1 -> Product_1e13a/2
  State_psi_q_SG_D_1_2f227/1 -> Add_41e5d/2
  Constant_-1_678d3/1 -> Product_90f35/1
  State_psi_1d_SG_D_1_f309e/1 -> Product_90f35/2
  Constant_x_ddd_8eddf/1 -> Subtract_f0ea0/2
  State_psi_gq_SG_D_1_d9ca3/1 -> Product_72354/1
  Add_8b435/1 -> Product_72354/2
  Product_f8e2c/1 -> Add_b16f4/1
  Product_444a5/1 -> Product_b7782/1
  Constant_x_qd_59921/1 -> Add_b16f4/2
  Product_a161f/1 -> Divide_f6ea0/1
  State_psi_kq_SG_D_1_0f8e3/1 -> Product_aae9b/1
  Add_b16f4/1 -> Divide_2779c/2
  Subtract_16297/1 -> Product_aae9b/2
  Product_28f44/1 -> Add_04fe2/1
  Constant_x_qd_2b014/1 -> Add_04fe2/2
  Product_aae9b/1 -> Divide_b9c05/1
  Product_90f35/1 -> Product_a161f/1
  Constant_x_dd_bd552/1 -> Subtract_50a5f/1
  Constant_x_l_aae67/1 -> Subtract_50a5f/2
  Constant_x_ddd_62423/1 -> Subtract_a62de/1
  Product_1e13a/1 -> Divide_7cbd0/1
  Constant_x_l_a8e7e/1 -> Subtract_a62de/2
  Divide_30c30/1 -> Add_cd29b/1
  Product_b7782/1 -> Divide_30c30/1
  Add_04fe2/1 -> Divide_b9c05/2
  Subtract_c749b/1 -> Add_41e5d/1
  Divide_b9c05/1 -> Subtract_c749b/2
  Subtract_50a5f/1 -> Divide_f6ea0/2
  State_psi_fd_SG_D_1_d1c10/1 -> Product_c89ea/1
  Constant_x_ddd_6a04f/1 -> Divide_7cbd0/2
  Subtract_a62de/1 -> Product_c89ea/2
  Constant_x_dd_10022/1 -> Subtract_37645/1
  Constant_x_l_4baef/1 -> Subtract_37645/2
  Divide_f6ea0/1 -> Add_7aebe/1
  Add_7aebe/1 -> Subtract_8cdf0/1
  State_psi_d_SG_D_1_8592d/1 -> Add_7aebe/2
  Product_c89ea/1 -> Divide_c5dbb/1
  Subtract_37645/1 -> Divide_c5dbb/2
  Constant_-1_fbcda/1 -> Product_444a5/1
  State_psi_d_SG_D_1_e2ff8/1 -> Product_444a5/2
  Divide_c5dbb/1 -> Subtract_8cdf0/2
  Add_41e5d/1 -> Product_b7782/2
  Divide_7cbd0/1 -> Add_cd29b/2
  Add_cd29b/1 -> Blockout_T_e_SG_D_1_2bf50/1

== system case6/SG_D_1/d_E_fd_SG_D_1_block ==
  note: d_E_fd_SG_D_1 in case6
      | $\frac{V_{f,\mathrm{SG},D,1}-E_{\mathrm{fd},\mathrm{SG},D,1}\,K_{E}}{T_{E}}$
      | Automatically generated on 2025-10-31 19:17:05 .
  State_E_fd_SG_D_1_82de9 : Inport
  State_V_f_SG_D_1_13d9b : Inport  Port=2
  Add_4bcbd : Sum
  Constant_-1_2f6b6 : Constant  Value=-1
  Constant_K_E_61218 : Constant  Value=K_E
  Constant_T_E_0a0bf : Constant  Value=T_E
  Divide_aa69a : Product  Inputs=*/
  Product_0190d : Product
  Product_d1124 : Product
  Blockout_d_E_fd_SG_D_1_37355 : Outport
  wires:
  Add_4bcbd/1 -> Divide_aa69a/1
  Constant_-1_2f6b6/1 -> Product_0190d/1
  State_E_fd_SG_D_1_82de9/1 -> Product_0190d/2
  Product_0190d/1 -> Product_d1124/1
  Constant_K_E_61218/1 -> Product_d1124/2
  Product_d1124/1 -> Add_4bcbd/1
  Constant_T_E_0a0bf/1 -> Divide_aa69a/2
  State_V_f_SG_D_1_13d9b/1 -> Add_4bcbd/2
  Divide_aa69a/1 -> Blockout_d_E_fd_SG_D_1_37355/1

== system case6/SG_D_1/d_Px_1_SG_D_1_block ==
  note: d_Px_1_SG_D_1 in case6
      | $\frac{w_{\mathrm{SG},D,1}-2\,\pi \,f_{0}}{T_{w}}-\frac{\mathrm{Px}_{1,\mathrm{SG},D,1}}{T_{w}}$
      | Automatically generated on 2025-10-31 19:17:06 .
  State_Px_1_SG_D_1_dc6c6 : Inport
  State_w_SG_D_1_eeef3 : Inport  Port=2
  Add_00600 : Sum
  Add_78a42 : Sum
  Constant_-1_fad26 : Constant  Value=-1
  Constant_-2.0_311eb : Constant  Value=-2.0
  Constant_T_w_637ec : Constant  Value=T_w
  Constant_T_w_cc975 : Constant  Value=T_w
  Constant_f0_2ca8d : Constant  Value=f0
  Constant_pi_e7d17 : Constant  Value=pi
  Divide_ab315 : Product  Inputs=*/
  Divide_ba724 : Product  Inputs=*/
  Product_1df40 : Product
  Product_a9083 : Product
  Product_bbbec : Product
  Blockout_d_Px_1_SG_D_1_0615f : Outport
  wires:
  Add_78a42/1 -> Blockout_d_Px_1_SG_D_1_0615f/1
  Constant_-2.0_311eb/1 -> Product_a9083/1
  Product_1df40/1 -> Divide_ab315/1
  State_w_SG_D_1_eeef3/1 -> Add_00600/2
  Constant_-1_fad26/1 -> Product_1df40/1
  Constant_f0_2ca8d/1 -> Product_bbbec/2
  Constant_pi_e7d17/1 -> Product_a9083/2
  Product_bbbec/1 -> Add_00600/1
  Product_a9083/1 -> Product_bbbec/1
  State_Px_1_SG_D_1_dc6c6/1 -> Product_1df40/2
  Constant_T_w_cc975/1 -> Divide_ab315/2
  Add_00600/1 -> Divide_ba724/1
  Constant_T_w_637ec/1 -> Divide_ba724/2
  Divide_ab315/1 -> Add_78a42/1
  Divide_ba724/1 -> Add_78a42/2

== system case6/SG_D_1/d_Px_2_SG_D_1_block ==
  note: d_Px_2_SG_D_1 in case6
      | $\frac{\mathrm{Px}_{1,\mathrm{SG},D,1}-T_{2}\,\left(\frac{\mathrm{Px}_{1,\mathrm{SG},D,1}}{T_{w}}-\frac{w_{\mathrm{SG},D,1}-2\,\pi \,f_{0}}{T_{w}}\right)}{T_{1}}-\frac{\mathrm{Px}_{2,\mathrm{SG},D,1}}{T_{1}}$
      | Automatically generated on 2025-10-31 19:17:08 .
  State_Px_2_SG_D_1_69c24 : Inport
  State_Px_1_SG_D_1_60b9a : Inport  Port=2
  State_Px_1_SG_D_1_da658 : Inport  Port=3
  State_w_SG_D_1_2ac36 : Inport  Port=4
  Add_00440 : Sum
  Add_4bb16 : Sum
  Add_84c23 : Sum
  Add_d6f5b : Sum
  Constant_-1_461b0 : Constant  Value=-1
  Constant_-1_73a68 : Constant  Value=-1
  Constant_-2.0_8cd9b : Constant  Value=-2.0
  Constant_T_1_32d98 : Constant  Value=T_1
  Constant_T_1_d38b2 : Constant  Value=T_1
  Constant_T_2_796e5 : Constant  Value=T_2
  Constant_T_w_60c4d : Constant  Value=T_w
  Constant_T_w_88125 : Constant  Value=T_w
  Constant_f0_e1d7f : Constant  Value=f0
  Constant_pi_35c78 : Constant  Value=pi
  Divide_01dce : Product  Inputs=*/
  Divide_6b01f : Product  Inputs=*/
  Divide_c2b02 : Product  Inputs=*/
  Divide_fe590 : Product  Inputs=*/
  Product_04f7f : Product
  Product_60135 : Product
  Product_90b7d : Product
  Product_c8392 : Product
  Product_e91e4 : Product
  Blockout_d_Px_2_SG_D_1_ff825 : Outport
  wires:
  Constant_-2.0_8cd9b/1 -> Product_04f7f/1
  State_w_SG_D_1_2ac36/1 -> Add_4bb16/2
  Constant_f0_e1d7f/1 -> Product_e91e4/2
  Constant_pi_35c78/1 -> Product_04f7f/2
  Add_84c23/1 -> Product_90b7d/2
  Product_e91e4/1 -> Add_4bb16/1
  Divide_fe590/1 -> Add_84c23/1
  Product_04f7f/1 -> Product_e91e4/1
  Constant_T_w_88125/1 -> Divide_fe590/2
  Constant_-1_73a68/1 -> Product_60135/1
  State_Px_1_SG_D_1_da658/1 -> Product_60135/2
  Divide_6b01f/1 -> Add_d6f5b/1
  Product_60135/1 -> Divide_fe590/1
  Add_4bb16/1 -> Divide_c2b02/1
  Constant_T_w_60c4d/1 -> Divide_c2b02/2
  Divide_c2b02/1 -> Add_84c23/2
  Constant_T_2_796e5/1 -> Product_90b7d/1
  Constant_-1_461b0/1 -> Product_c8392/1
  State_Px_2_SG_D_1_69c24/1 -> Product_c8392/2
  State_Px_1_SG_D_1_60b9a/1 -> Add_00440/1
  Product_90b7d/1 -> Add_00440/2
  Add_00440/1 -> Divide_01dce/1
  Product_c8392/1 -> Divide_6b01f/1
  Constant_T_1_32d98/1 -> Divide_6b01f/2
  Constant_T_1_d38b2/1 -> Divide_01dce/2
  Divide_01dce/1 -> Add_d6f5b/2
  Add_d6f5b/1 -> Blockout_d_Px_2_SG_D_1_ff825/1

== system case6/SG_D_1/d_Px_3_SG_D_1_block ==
  note: d_Px_3_SG_D_1 in case6
      | $\frac{\mathrm{Px}_{2,\mathrm{SG},D,1}+T_{4}\,\left(\frac{\mathrm{Px}_{1,\mathrm{SG},D,1}-T_{2}\,\left(\frac{\mathrm{Px}_{1,\mathrm{SG},D,1}}{T_{w}}-\frac{w_{\mathrm{SG},D,1}-2\,\pi \,f_{0}}{T_{w}}\right)}{T_{1}}-\frac{\mathrm{Px}_{2,\mathrm{SG},D,1}}{T_{1}}\right)}{T_{3}}-\frac{\mathrm{Px}_{3,\mathrm{SG},D,1}}{T_{3}}$
      | Automatically generated on 2025-10-31 19:17:10 .
  State_Px_3_SG_D_1_4b68a : Inport
  State_Px_2_SG_D_1_a88ed : Inport  Port=2
  State_Px_2_SG_D_1_521c0 : Inport  Port=3
  State_Px_1_SG_D_1_9c2b8 : Inport  Port=4
  State_Px_1_SG_D_1_097d2 : Inport  Port=5
  State_w_SG_D_1_3feaa : Inport  Port=6
  Add_1ee91 : Sum
  Add_2a88d : Sum
  Add_34b09 : Sum
  Add_75f52 : Sum
  Add_99153 : Sum
  Add_9fcf4 : Sum
  Constant_-1_28f89 : Constant  Value=-1
  Constant_-1_899b8 : Constant  Value=-1
  Constant_-1_8b889 : Constant  Value=-1
  Constant_-2.0_2744c : Constant  Value=-2.0
  Constant_T_1_5c185 : Constant  Value=T_1
  Constant_T_1_ef15f : Constant  Value=T_1
  Constant_T_2_c637d : Constant  Value=T_2
  Constant_T_3_1c4bc : Constant  Value=T_3
  Constant_T_3_cde6f : Constant  Value=T_3
  Constant_T_4_f4c25 : Constant  Value=T_4
  Constant_T_w_57c27 : Constant  Value=T_w
  Constant_T_w_b4efa : Constant  Value=T_w
  Constant_f0_b9bae : Constant  Value=f0
  Constant_pi_e0d88 : Constant  Value=pi
  Divide_13b7d : Product  Inputs=*/
  Divide_1f07b : Product  Inputs=*/
  Divide_59d7d : Product  Inputs=*/
  Divide_a5ff8 : Product  Inputs=*/
  Divide_e228c : Product  Inputs=*/
  Divide_f3b6b : Product  Inputs=*/
  Product_33b04 : Product
  Product_6bf25 : Product
  Product_8c28c : Product
  Product_9d664 : Product
  Product_a6b06 : Product
  Product_a8900 : Product
  Product_d914c : Product
  Blockout_d_Px_3_SG_D_1_10237 : Outport
  wires:
  Constant_T_w_b4efa/1 -> Divide_13b7d/2
  Constant_-1_28f89/1 -> Product_33b04/1
  Add_99153/1 -> Blockout_d_Px_3_SG_D_1_10237/1
  Constant_-2.0_2744c/1 -> Product_8c28c/1
  State_w_SG_D_1_3feaa/1 -> Add_1ee91/2
  Constant_f0_b9bae/1 -> Product_d914c/2
  State_Px_1_SG_D_1_097d2/1 -> Product_33b04/2
  Constant_pi_e0d88/1 -> Product_8c28c/2
  Product_d914c/1 -> Add_1ee91/1
  Product_8c28c/1 -> Product_d914c/1
  Product_33b04/1 -> Divide_13b7d/1
  Divide_e228c/1 -> Add_99153/1
  Constant_T_3_cde6f/1 -> Divide_a5ff8/2
  Add_1ee91/1 -> Divide_f3b6b/1
  Constant_T_w_57c27/1 -> Divide_f3b6b/2
  Divide_13b7d/1 -> Add_34b09/1
  Divide_f3b6b/1 -> Add_34b09/2
  Constant_-1_899b8/1 -> Product_a8900/1
  Constant_T_2_c637d/1 -> Product_a6b06/1
  Add_34b09/1 -> Product_a6b06/2
  Constant_-1_8b889/1 -> Product_9d664/1
  Divide_a5ff8/1 -> Add_99153/2
  Constant_T_3_1c4bc/1 -> Divide_e228c/2
  State_Px_2_SG_D_1_521c0/1 -> Product_9d664/2
  State_Px_1_SG_D_1_9c2b8/1 -> Add_9fcf4/1
  Divide_1f07b/1 -> Add_75f52/1
  Product_a6b06/1 -> Add_9fcf4/2
  Product_9d664/1 -> Divide_1f07b/1
  Product_a8900/1 -> Divide_e228c/1
  Constant_T_1_ef15f/1 -> Divide_1f07b/2
  Add_9fcf4/1 -> Divide_59d7d/1
  Constant_T_1_5c185/1 -> Divide_59d7d/2
  Divide_59d7d/1 -> Add_75f52/2
  Constant_T_4_f4c25/1 -> Product_6bf25/1
  Add_75f52/1 -> Product_6bf25/2
  State_Px_3_SG_D_1_4b68a/1 -> Product_a8900/2
  State_Px_2_SG_D_1_a88ed/1 -> Add_2a88d/1
  Product_6bf25/1 -> Add_2a88d/2
  Add_2a88d/1 -> Divide_a5ff8/1

== system case6/SG_D_1/d_R_f_SG_D_1_block ==
  note: d_R_f_SG_D_1 in case6
      | $-\frac{R_{f,\mathrm{SG},D,1}-\frac{E_{\mathrm{fd},\mathrm{SG},D,1}\,K_{F}}{T_{F}}}{T_{F}}$
      | Automatically generated on 2025-10-31 19:17:04 .
  State_E_fd_SG_D_1_af68a : Inport
  State_R_f_SG_D_1_dba0c : Inport  Port=2
  Constant_K_F_a4f27 : Constant  Value=K_F
  Constant_T_F_9908e : Constant  Value=T_F
  Constant_T_F_a8c8c : Constant  Value=T_F
  Divide_afe1d : Product  Inputs=*/
  Divide_b3aa3 : Product  Inputs=*/
  Product_b6913 : Product
  Subtract_dc129 : Sum  Inputs=+-
  Blockout_d_R_f_SG_D_1_5dd2e : Outport
  wires:
  Constant_K_F_a4f27/1 -> Product_b6913/2
  Product_b6913/1 -> Divide_b3aa3/1
  State_E_fd_SG_D_1_af68a/1 -> Product_b6913/1
  State_R_f_SG_D_1_dba0c/1 -> Subtract_dc129/2
  Constant_T_F_9908e/1 -> Divide_b3aa3/2
  Divide_b3aa3/1 -> Subtract_dc129/1
  Divide_afe1d/1 -> Blockout_d_R_f_SG_D_1_5dd2e/1
  Subtract_dc129/1 -> Divide_afe1d/1
  Constant_T_F_a8c8c/1 -> Divide_afe1d/2

== system case6/SG_D_1/d_T_m_SG_D_1_block ==
  note: d_T_m_SG_D_1 in case6
      | $-\frac{T_{m,\mathrm{SG},D,1}-T_{0}+\frac{\mathrm{SpeedPara}\,\left(w_{\mathrm{SG},D,1}-w_{\mathrm{ref}}\right)}{2\,f_{0}\,\pi }}{T_{\mathrm{speed}}}$
      | Automatically generated on 2025-10-31 19:16:55 .
  State_w_SG_D_1_3ea60 : Inport
  State_T_m_SG_D_1_5ba5d : Inport  Port=2
  Add_dda79 : Sum
  Add_f727b : Sum
  Constant_-1_8974d : Constant  Value=-1
  Constant_2.0_dcd68 : Constant  Value=2.0
  Constant_SpeedPara_317d2 : Constant  Value=SpeedPara
  Constant_T_0_67c96 : Constant  Value=T_0
  Constant_T_speed_39fb2 : Constant  Value=T_speed
  Constant_f0_f4b3c : Constant  Value=f0
  Constant_pi_fdc2a : Constant  Value=pi
  Constant_w_ref_069c4 : Constant  Value=w_ref
  Divide_2fc41 : Product  Inputs=*/
  Divide_43e43 : Product  Inputs=*/
  Product_42e02 : Product
  Product_c4c04 : Product
  Product_ce5f6 : Product
  Product_f6ff9 : Product
  Subtract_0209b : Sum  Inputs=+-
  Blockout_d_T_m_SG_D_1_63317 : Outport
  wires:
  Constant_-1_8974d/1 -> Product_c4c04/1
  Constant_w_ref_069c4/1 -> Add_f727b/2
  State_w_SG_D_1_3ea60/1 -> Product_c4c04/2
  Add_dda79/1 -> Subtract_0209b/1
  Add_f727b/1 -> Product_42e02/2
  Product_c4c04/1 -> Add_f727b/1
  Constant_2.0_dcd68/1 -> Product_ce5f6/1
  Constant_pi_fdc2a/1 -> Product_ce5f6/2
  Constant_SpeedPara_317d2/1 -> Product_42e02/1
  Product_ce5f6/1 -> Product_f6ff9/1
  Constant_f0_f4b3c/1 -> Product_f6ff9/2
  Constant_T_speed_39fb2/1 -> Divide_43e43/2
  Product_42e02/1 -> Divide_2fc41/1
  Product_f6ff9/1 -> Divide_2fc41/2
  Divide_2fc41/1 -> Add_dda79/1
  Constant_T_0_67c96/1 -> Add_dda79/2
  State_T_m_SG_D_1_5ba5d/1 -> Subtract_0209b/2
  Subtract_0209b/1 -> Divide_43e43/1
  Divide_43e43/1 -> Blockout_d_T_m_SG_D_1_63317/1
